simulink model "test"  (R2015a)
settings: Solver=ode45  StartTime=0.0  StopTime=200  RelTol=1e-3
libraries: simulink x1
settings Model: Creator=marco  LastModifiedBy=marco

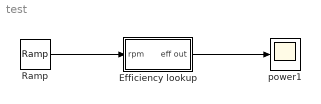
== system test ==
  Efficiency lookup : Subsystem
  Ramp : simulink/Sources/Ramp  slope=1  start=0  X0=0
  power1 : Scope
      settings: TimeRange=700  YMin=0  YMax=550  SaveName=ScopeData7  MaxDataPoints=scope_history
  wires:
  Efficiency lookup/1(eff out) -> power1/1
  Ramp/1 -> Efficiency lookup/1("rpm ")

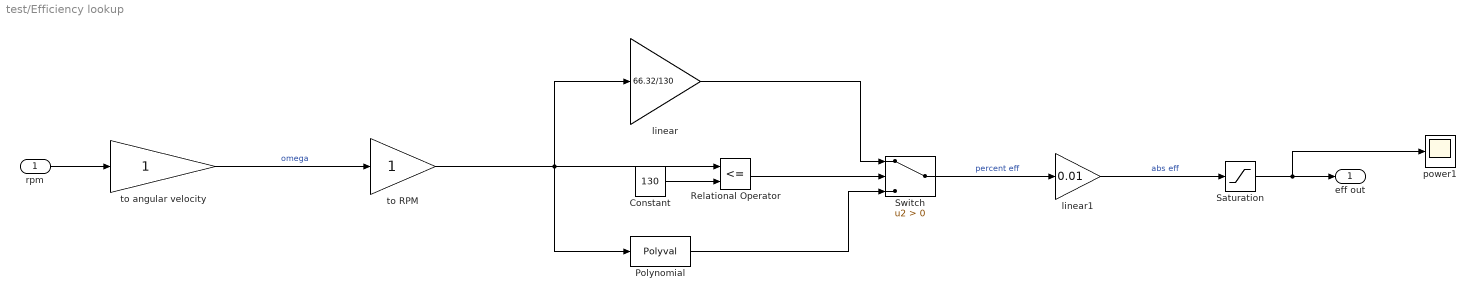
== system test/Efficiency lookup ==
  "rpm " : Inport
  Constant : Constant  Value=130
  Polynomial : Polyval  Coefs="[-0.000000281154604 0.00025333618 -0.0949601636 18.9528272 -2124.26186  126769.071 -3146791.96]"
  Relational Operator : RelationalOperator  Operator=<=  OutDataTypeStr=boolean
  Saturation : Saturate  UpperLimit=1  LowerLimit=0.05
  Switch : Switch  Criteria=u2 > Threshold
  linear : Gain  Gain=66.32/130
  linear1 : Gain  Gain=0.01
  power1 : Scope
      settings: TimeRange=700  YMin=0  YMax=140  SaveName=ScopeData13  MaxDataPoints=scope_history
  to RPM : Gain
  to angular velocity : Gain
  eff out : Outport
  wires:
  "rpm "/1 -> to angular velocity/1
  to angular velocity/1 -> to RPM/1  "omega"
  Constant/1 -> Relational Operator/2
  Relational Operator/1 -> Switch/2
  Polynomial/1 -> Switch/3
  linear/1 -> Switch/1
  linear1/1 -> Saturation/1  "abs eff"
  Saturation/1 -> power1/1, eff out/1
  to RPM/1 -> Polynomial/1, linear/1, Relational Operator/1
  Switch/1 -> linear1/1  "percent eff"
